simulink model "RCAI_ControlsSimulinkModel"  (R2019b)
settings: Solver=FixedStepAuto  StartTime=0.0  StopTime=inf  FixedStep=0.025  RelTol=1e-3
undefined symbols (not defined in the file): Header, Seq, Stamp, Vector_
libraries: robotlib x5, simulink x1, robotmobilelib x1
settings Model: Creator=The MathWorks, Inc.  LastModifiedBy=pmeautonomy
settings OptimizationCC: EnhancedBackFolding=on  PassReuseOutputArgsAs=Individual arguments  ZeroExternalMemoryAtStartup=off  ZeroInternalMemoryAtStartup=off  MaxStackSize=64  OptimizeBlockOrder=speed  DifferentSizesBufferReuse=on  OptimizationCustomize=off  EfficientTunableParamExpr=on
settings DebuggingCC: ParameterTunabilityLossMsg=error
settings HardwareCC: ProdBitPerLong=64  ProdHWDeviceType=Intel->x86-64 (Linux 64)
settings SFSimCC: MATLABDynamicMemAlloc=off
settings RTWCC: SystemTargetFile=ert.tlc  HardwareBoard=Robot Operating System (ROS)  TLCOptions="-aInlineSetEventsForThisBaseRateFcn=TLC_FALSE -aSuppressMultiTaskScheduler=TLC_FALSE  -aRateBasedStepFcn=0"  TemplateMakefile=ert_default_tmf  GenerateReport=on  Toolchain=Catkin  IncludeHyperlinkInReport=on  LaunchReport=on  TargetLang=C++  GenerateTraceInfo=on  GenerateTraceReport=on  GenerateTraceReportSl=on  GenerateTraceReportSf=on  GenerateTraceReportEml=on
settings CodeAppCC: ForceParamTrailComments=on  IgnoreCustomStorageClasses=off  OperatorAnnotations=on  SimulinkDataObjDesc=on  SFDataObjDesc=on  InsertBlockDesc=on

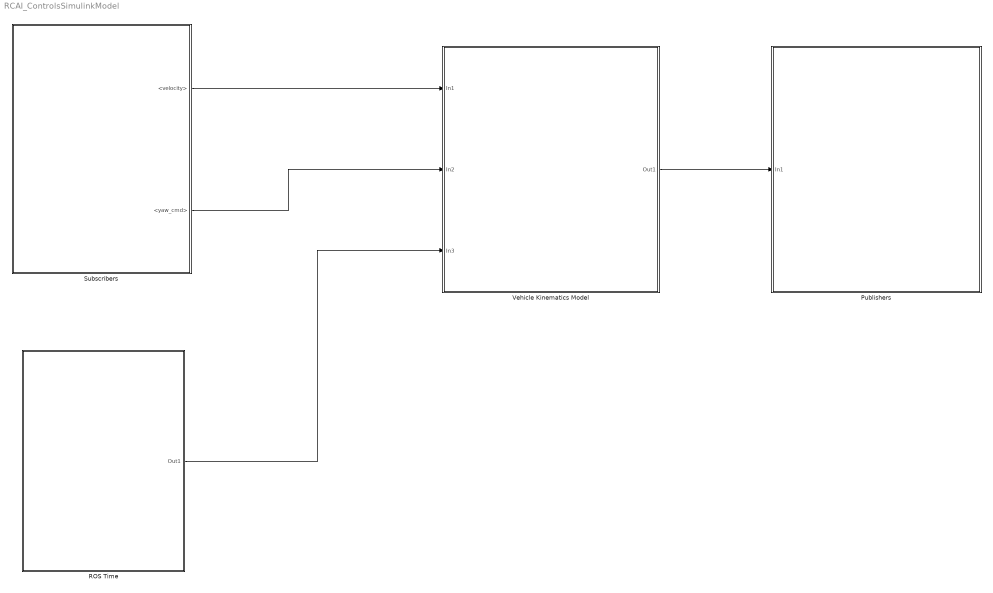
== system RCAI_ControlsSimulinkModel ==
  Publishers : Subsystem
  ROS Time : Subsystem
  Subscribers : Subsystem
  Vehicle Kinematics Model : Subsystem
  wires:
  Subscribers/1(<velocity>) -> Vehicle Kinematics Model/1(In1)
  Subscribers/2(<yaw_cmd>) -> Vehicle Kinematics Model/2(In2)
  Vehicle Kinematics Model/1(Out1) -> Publishers/1(In1)
  ROS Time/1(Out1) -> Vehicle Kinematics Model/3(In3)

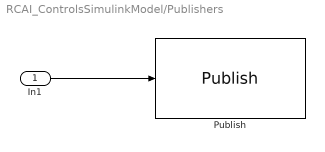
== system RCAI_ControlsSimulinkModel/Publishers ==
  In1 : Inport
  Publish : robotlib/Publish  topicSource=Specify your own  topic=/vehicle_dynamics  messageType=geometry_msgs/Vector3Stamped  messageQueueLength=1
      settings: SourceProductName=ROS Toolbox
  wires:
  In1/1 -> Publish/1

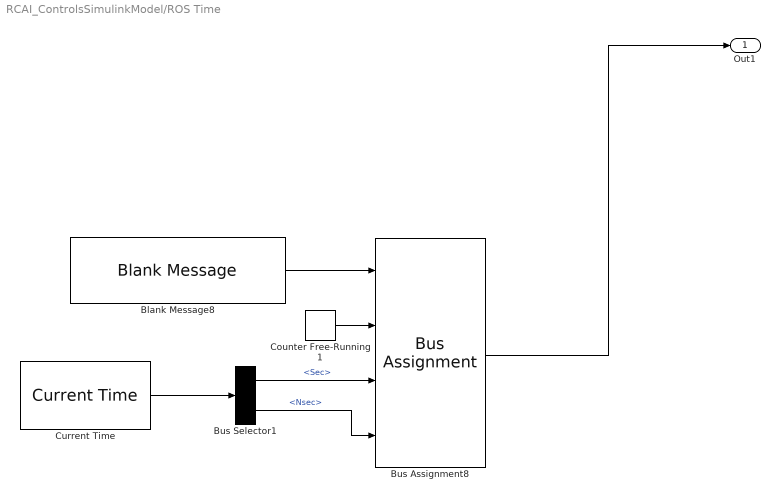
== system RCAI_ControlsSimulinkModel/ROS Time ==
  Blank Message8 : robotlib/Blank Message  messageClass=Message  entityType=std_msgs/Header  messageType=std_msgs/Header  SampleTime=inf
      settings: SourceProductBaseCode=RO
  Bus Assignment8 : BusAssignment  AssignedSignals=Seq,Stamp.Sec,Stamp.Nsec
  Bus Selector1 : BusSelector  OutputSignals=Sec,Nsec
  Counter Free-Running1 : simulink/Sources/Counter Free-Running  NumBits=32  tsamp=-1
  Current Time : robotlib/Current Time  OutputFormat=bus  SampleTime=-1  ModelName=RCAI_ControlsSimulinkModel
      settings: SourceProductName=ROS Toolbox  SourceProductBaseCode=RR
  Out1 : Outport
  wires:
  Counter Free-Running1/1 -> Bus Assignment8/2
  Bus Selector1/2 -> Bus Assignment8/4  "<Nsec>"
  Blank Message8/1 -> Bus Assignment8/1
  Bus Selector1/1 -> Bus Assignment8/3  "<Sec>"
  Current Time/1 -> Bus Selector1/1
  Bus Assignment8/1 -> Out1/1

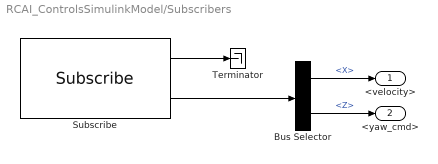
== system RCAI_ControlsSimulinkModel/Subscribers ==
  Bus Selector : BusSelector  OutputSignals=Twist.Linear.X,Twist.Angular.Z
  Subscribe : robotlib/Subscribe  topicSource=Specify your own  topic=/MobilityCmd  messageType=geometry_msgs/TwistStamped  sampleTime=-1  messageQueueLength=1
      settings: SourceProductName=ROS Toolbox
  Terminator : Terminator
  <velocity> : Outport
  <yaw_cmd> : Outport  Port=2
  wires:
  Subscribe/1 -> Terminator/1
  Bus Selector/1 -> <velocity>/1  "<X>"
  Subscribe/2 -> Bus Selector/1
  Bus Selector/2 -> <yaw_cmd>/1  "<Z>"

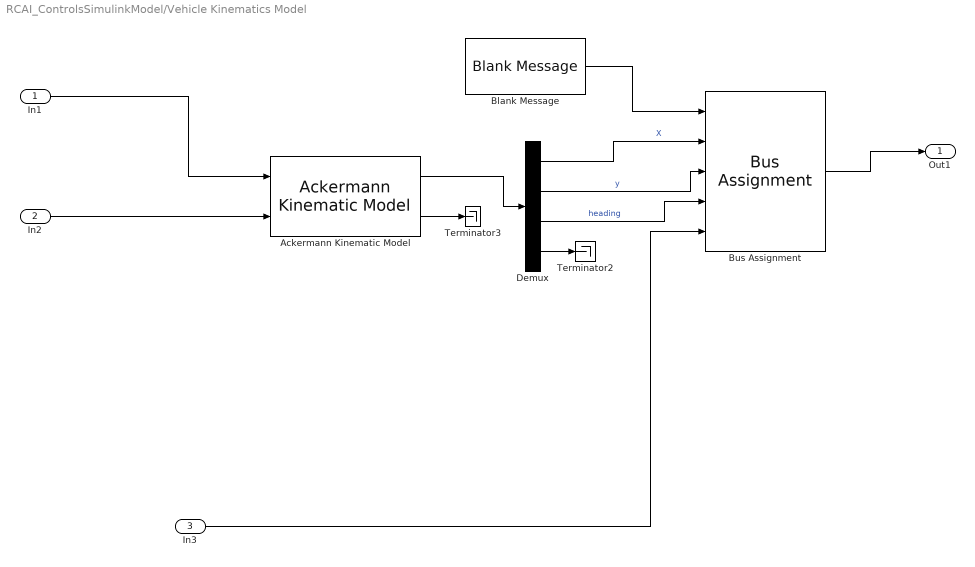
== system RCAI_ControlsSimulinkModel/Vehicle Kinematics Model ==
  In1 : Inport
  In2 : Inport  Port=2
  In3 : Inport  Port=3
  Ackermann Kinematic Model : robotmobilelib/Ackermann Kinematic Model  WheelBase=3.089  VehicleSpeedRange=[-20 50]  MaxSteeringAngle=pi/4  InitialState=[0; 0; 0; 0]  SimulateUsing=Interpreted execution
      settings: SourceProductName=Robotics System Toolbox  SourceProductBaseCode=RO
  Blank Message : robotlib/Blank Message  messageClass=Message  entityType=geometry_msgs/Vector3Stamped  messageType=geometry_msgs/Vector3Stamped  SampleTime=inf
      settings: SourceProductName=ROS Toolbox
  Bus Assignment : BusAssignment  AssignedSignals=Vector_.X,Vector_.Y,Vector_.Z,Header
  Demux : Demux
  Terminator2 : Terminator
  Terminator3 : Terminator
  Out1 : Outport
  wires:
  Bus Assignment/1 -> Out1/1
  Ackermann Kinematic Model/1 -> Demux/1
  Blank Message/1 -> Bus Assignment/1
  Ackermann Kinematic Model/2 -> Terminator3/1
  In2/1 -> Ackermann Kinematic Model/2
  Demux/2 -> Bus Assignment/3  "y"
  In3/1 -> Bus Assignment/5
  Demux/3 -> Bus Assignment/4  "heading"
  Demux/4 -> Terminator2/1
  In1/1 -> Ackermann Kinematic Model/1
  Demux/1 -> Bus Assignment/2  "X"
